simulink model "instruction_memory"  (R2025b)
settings: Solver=VariableStepAuto  StartTime=0.0  StopTime=10.0  RelTol=1e-3
settings Model: Creator=cyber  LastModifiedBy=cyber

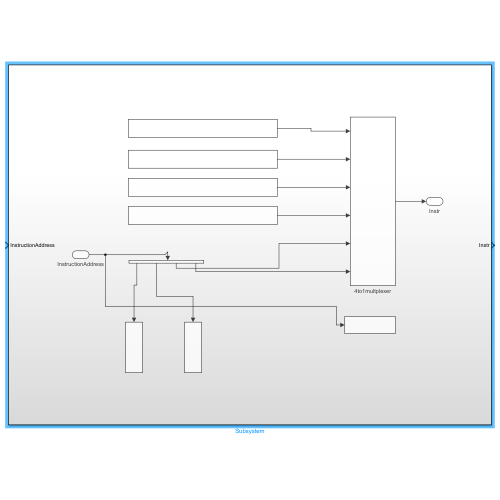
[thumbnail: Simulink's stored preview of the top-level diagram]
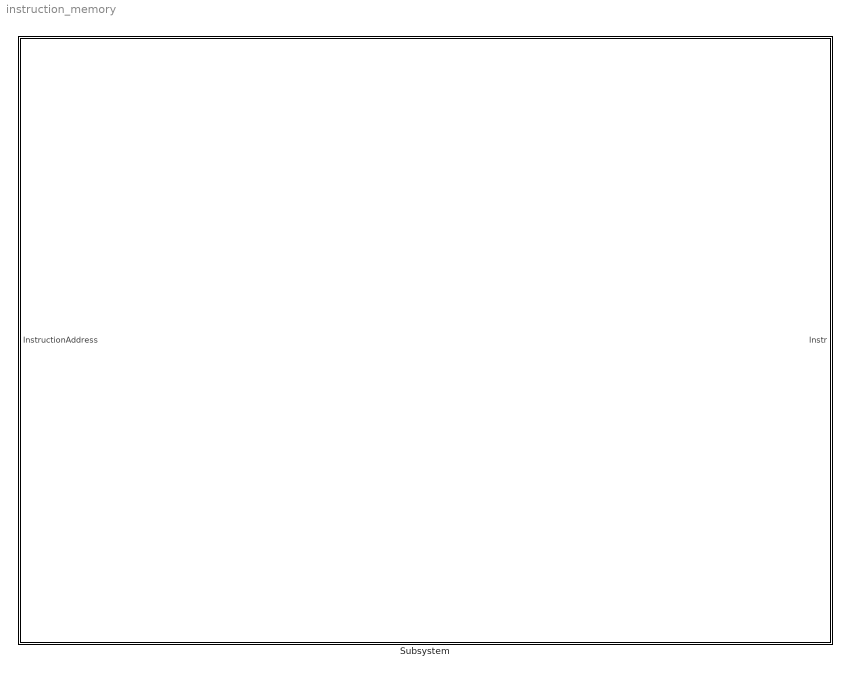
== system instruction_memory ==
  Subsystem : Subsystem

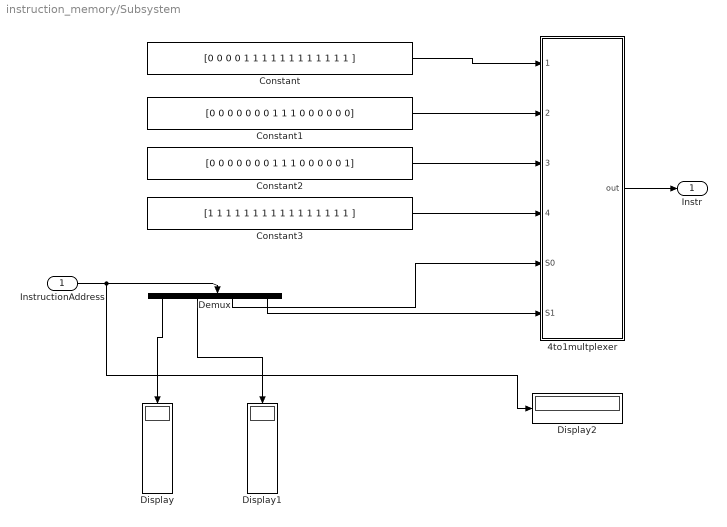
== system instruction_memory/Subsystem ==
  InstructionAddress : Inport
  4to1multplexer : Subsystem
  Constant : Constant  Value=[0 0 0 0 1 1 1 1 1 1 1 1 1 1 1 1 ]
  Constant1 : Constant  Value=[0 0 0 0 0 0 0 1 1 1 0 0 0 0 0 0]
  Constant2 : Constant  Value=[0 0 0 0 0 0 0 1 1 1 0 0 0 0 0 1]
  Constant3 : Constant  Value=[1 1 1 1 1 1 1 1 1 1 1 1 1 1 1 1 ]
  Demux : Demux
  Display : Display
  Display1 : Display
  Display2 : Display
  Instr : Outport
  wires:
  Demux/3 -> 4to1multplexer/5(S0)
  Demux/2 -> Display1/1
  Constant1/1 -> 4to1multplexer/2(2)
  Constant3/1 -> 4to1multplexer/4(4)
  Constant/1 -> 4to1multplexer/1(1)
  4to1multplexer/1(out) -> Instr/1
  Demux/4 -> 4to1multplexer/6(S1)
  Constant2/1 -> 4to1multplexer/3(3)
  InstructionAddress/1 -> Demux/1, Display2/1
  Demux/1 -> Display/1

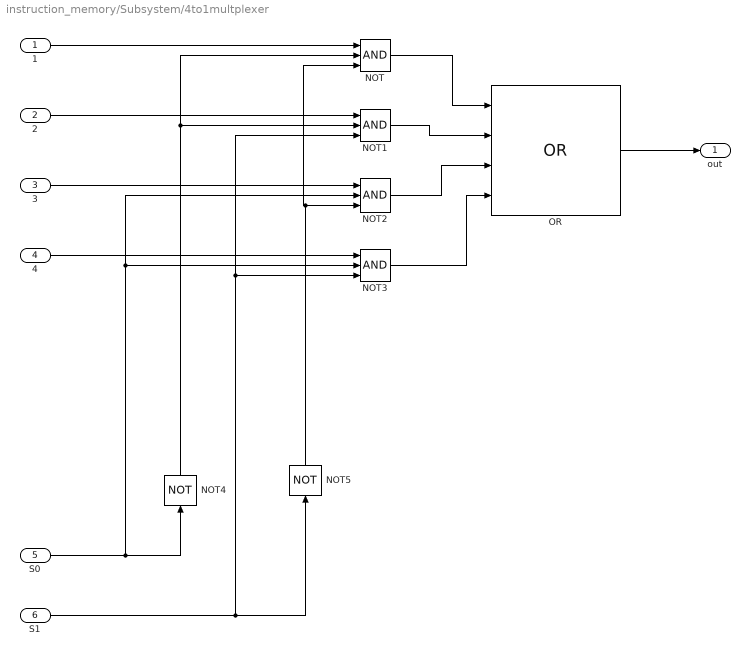
== system instruction_memory/Subsystem/4to1multplexer ==
  1 : Inport
  2 : Inport  Port=2
  3 : Inport  Port=3
  4 : Inport  Port=4
  S0 : Inport  Port=5
  S1 : Inport  Port=6
  NOT{,1..3} (4 alike) : Logic  Inputs=3  IconShape=distinctive  AllPortsSameDT=off  OutDataTypeStr=boolean
  NOT4 : Logic  Operator=NOT  IconShape=distinctive  AllPortsSameDT=off  OutDataTypeStr=boolean
  NOT5 : Logic  Operator=NOT  IconShape=distinctive  AllPortsSameDT=off  OutDataTypeStr=boolean
  OR : Logic  Operator=OR  Inputs=4  IconShape=distinctive  AllPortsSameDT=off  OutDataTypeStr=boolean
  out : Outport
  wires:
  NOT4/1 -> NOT/2, NOT1/2
  S1/1 -> NOT1/3, NOT3/3, NOT5/1
  NOT5/1 -> NOT/3, NOT2/3
  NOT1/1 -> OR/2
  S0/1 -> NOT4/1, NOT3/2, NOT2/2
  NOT3/1 -> OR/4
  NOT/1 -> OR/1
  NOT2/1 -> OR/3
  4/1 -> NOT3/1
  1/1 -> NOT/1
  3/1 -> NOT2/1
  2/1 -> NOT1/1
  OR/1 -> out/1
